simulink model "sim_simulink1"  (R2019a)
settings: Solver=VariableStepAuto  StartTime=0.0  StopTime=50.0  RelTol=1e-3
values from neighbouring files (symbols this model uses):
  kc = x(1)    [PID_IAE.m]    (also in PID_ISE.m; PID_ITAE.m; PID_ITSE.m; PI_IAE.m)
  td = x(3)    [PID_IAE.m]    (also in PID_ISE.m; PID_ITAE.m; PID_ITSE.m; PI_IAE.m = 0)
  ti = x(2)    [PID_IAE.m]    (also in PID_ISE.m; PID_ITAE.m; PID_ITSE.m; PI_IAE.m)
settings Model: Creator=gambi  LastModifiedBy=julio
settings DataIOCC: ReturnWorkspaceOutputs=off
settings DebuggingCC: ArithmeticOperatorsInVariantConditions=warning

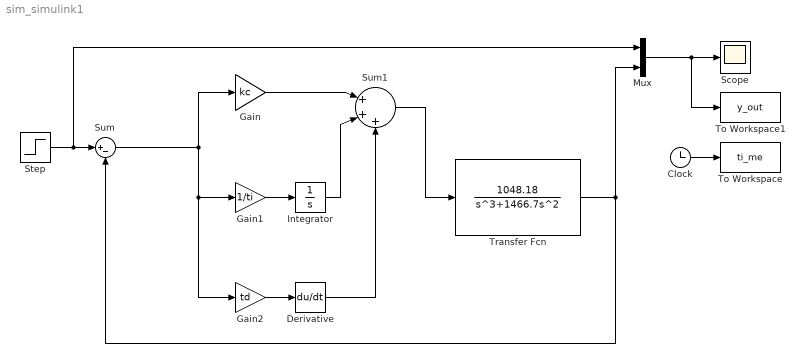
== system sim_simulink1 ==
  Clock : Clock
      settings: Decimation=30
  Derivative : Derivative
  Gain : Gain  Gain=kc
  Gain1 : Gain  Gain=1/ti
  Gain2 : Gain  Gain=td
  Integrator : Integrator
  Mux : Mux  Inputs=2
  Scope : Scope
  Step : Step  Time=0  SampleTime=0
  Sum : Sum  Inputs=|+-
  Sum1 : Sum  Inputs=|+++
  To Workspace : ToWorkspace  VariableName=ti_me  SampleTime=-1
  To Workspace1 : ToWorkspace  VariableName=y_out  SampleTime=-1
  Transfer Fcn : TransferFcn  Numerator=[1048.18]  Denominator=[1 1466.7 0 0]
  wires:
  Step/1 -> Mux/1, Sum/1
  Gain1/1 -> Integrator/1
  Gain2/1 -> Derivative/1
  Integrator/1 -> Sum1/2
  Derivative/1 -> Sum1/3
  Transfer Fcn/1 -> Sum/2, Mux/2
  Mux/1 -> To Workspace1/1, Scope/1
  Clock/1 -> To Workspace/1
  Sum1/1 -> Transfer Fcn/1
  Gain/1 -> Sum1/1
  Sum/1 -> Gain2/1, Gain1/1, Gain/1
